simulink model "solar_tracker"  (R2014a)
settings: Solver=ode45  StartTime=0.0  StopTime=10.0  RelTol=1e-3
libraries: simulink x1
settings Model: Creator=naina  LastModifiedBy=naina

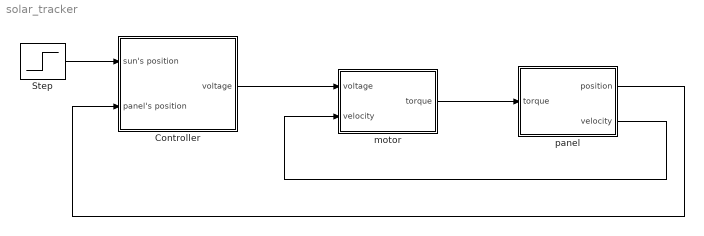
== system solar_tracker ==
  Controller : Subsystem
  Step : Step  SampleTime=0
  motor : Subsystem
  "panel " : Subsystem
  wires:
  "panel "/1("position ") -> Controller/2(panel's position)
  "panel "/2("velocity ") -> motor/2("velocity ")
  motor/1(torque) -> "panel "/1(torque)
  Step/1 -> Controller/1(sun's position)
  Controller/1(voltage) -> motor/1(voltage)

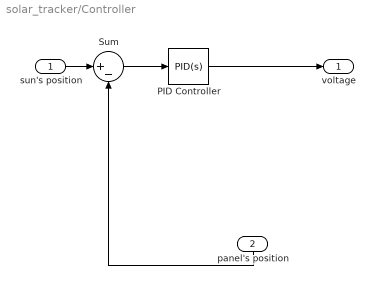
== system solar_tracker/Controller ==
  sun's position : Inport
  panel's position : Inport  Port=2
  PID Controller : simulink/Continuous/PID Controller  Controller=PID  TimeDomain=Continuous-time  SampleTime=1  IntegratorMethod=Forward Euler  FilterMethod=Forward Euler  Form=Parallel  P=1  I=1  D=0  N=100  InitialConditionSource=internal  InitialConditionForIntegrator=0  InitialConditionForFilter=0  ExternalReset=none  LimitOutput=off  UpperSaturationLimit=inf  LowerSaturationLimit=-inf  LinearizeAsGain=on  AntiWindupMode=none  Kb=1  TrackingMode=off  Kt=1  PParamMin=[]  PParamMax=[]  IParamMin=[]  IParamMax=[]  DParamMin=[]  DParamMax=[]  NParamMin=[]  NParamMax=[]  KbParamMin=[]  KbParamMax=[]  KtParamMin=[]  KtParamMax=[]  POutMin=[]  POutMax=[]  IOutMin=[]  IOutMax=[]  DOutMin=[]  DOutMax=[]  NOutMin=[]  NOutMax=[]  KbOutMin=[]  KbOutMax=[]  KtOutMin=[]  KtOutMax=[]  IntegratorOutMin=[]  IntegratorOutMax=[]  FilterOutMin=[]  FilterOutMax=[]  SumOutMin=[]  SumOutMax=[]  SumI1OutMin=[]  SumI1OutMax=[]  SumI2OutMin=[]  SumI2OutMax=[]  SumI3OutMin=[]  SumI3OutMax=[]  SumDOutMin=[]  SumDOutMax=[]  SaturationOutMin=[]  SaturationOutMax=[]  IntegratorContinuousStateAttributes=''  IntegratorStateMustResolveToSignalObject=off  IntegratorRTWStateStorageClass=Auto  FilterContinuousStateAttributes=''  FilterStateMustResolveToSignalObject=off  FilterRTWStateStorageClass=Auto
  Sum : Sum  Inputs=|+-
  voltage : Outport
  wires:
  sun's position/1 -> Sum/1
  panel's position/1 -> Sum/2
  PID Controller/1 -> voltage/1
  Sum/1 -> PID Controller/1

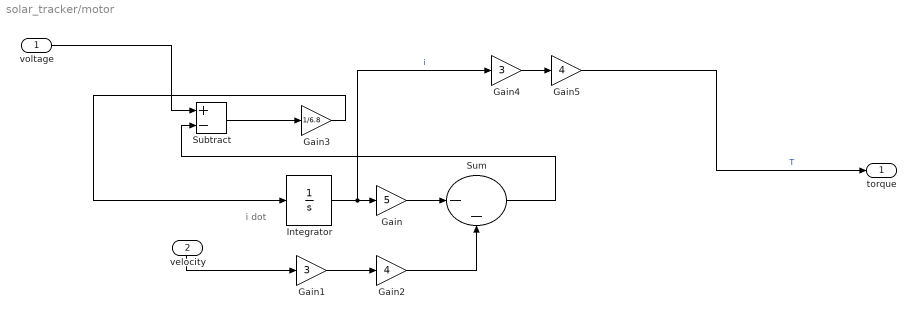
== system solar_tracker/motor ==
  note: i dot
  voltage : Inport
  "velocity " : Inport  Port=2
  Gain : Gain  Gain=5
  Gain1 : Gain  Gain=3
  Gain2 : Gain  Gain=4
  Gain3 : Gain  Gain=1/6.8
  Gain4 : Gain  Gain=3
  Gain5 : Gain  Gain=4
  Integrator : Integrator
  Subtract : Sum  Inputs=+-
  Sum : Sum  Inputs=|--
  torque : Outport
  wires:
  Integrator/1 -> Gain4/1, Gain/1  "i"
  Gain3/1 -> Integrator/1
  Gain2/1 -> Sum/2
  Gain1/1 -> Gain2/1
  Sum/1 -> Subtract/2
  Gain/1 -> Sum/1
  Gain5/1 -> torque/1  "T"
  "velocity "/1 -> Gain1/1
  Gain4/1 -> Gain5/1
  Subtract/1 -> Gain3/1
  voltage/1 -> Subtract/1

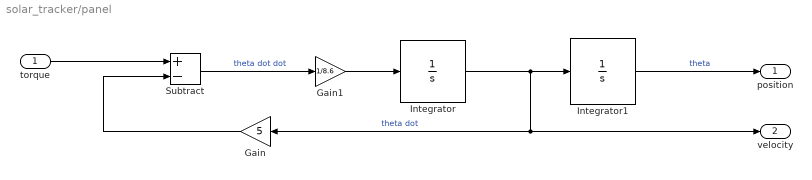
== system solar_tracker/panel  ==
  torque : Inport
  Gain : Gain  Gain=5
  Gain1 : Gain  Gain=1/8.6
  Integrator : Integrator
  Integrator1 : Integrator
  Subtract : Sum  Inputs=+-
  "position " : Outport
  "velocity " : Outport  Port=2
  wires:
  Integrator1/1 -> "position "/1  "theta"
  Integrator/1 -> "velocity "/1, Gain/1, Integrator1/1  "theta dot"
  Subtract/1 -> Gain1/1  "theta dot dot"
  Gain1/1 -> Integrator/1
  torque/1 -> Subtract/1
  Gain/1 -> Subtract/2
